simulink model "U2"  (R2021a)
settings: Solver=VariableStepAuto  StartTime=0.0  StopTime=100  RelTol=1e-3
libraries: cstblocks x2
settings Model: Creator=wilso  LastModifiedBy=wilso

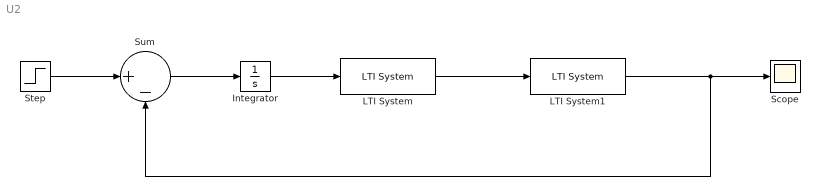
== system U2 ==
  Integrator : Integrator
  LTI System : cstblocks/LTI System  sys=c  IC=[]
  LTI System1 : cstblocks/LTI System  sys=G2  IC=[]
  Scope : Scope
  Step : Step  SampleTime=0
  Sum : Sum  Inputs=|+-
  wires:
  Integrator/1 -> LTI System/1
  Sum/1 -> Integrator/1
  LTI System/1 -> LTI System1/1
  LTI System1/1 -> Scope/1, Sum/2
  Step/1 -> Sum/1
